simulink model "collagenSim"  (R2021b)
settings: Solver=VariableStepAuto  StartTime=0.0  StopTime=900  RelTol=1e-3
libraries: fl_lib x360, nesl_utility x174, rllib x1
(part 1 of 4)
settings Model: SimulationMode=accelerator  Creator=Genis  LastModifiedBy=Genis
settings SolverCC: ZeroCrossAlgorithm=Adaptive  DecoupledContinuousIntegration=on
settings DebuggingCC: ReadBeforeWriteMsg=DisableAll  WriteAfterWriteMsg=DisableAll  WriteAfterReadMsg=DisableAll  IgnoredZcDiagnostic=none  MultiTaskDSMMsg=none  UnitsInconsistencyMsg=none
settings ModelReferenceCC: UpdateModelReferenceTargets=IfOutOfDate
settings SFSimCC: SFSimEcho=off

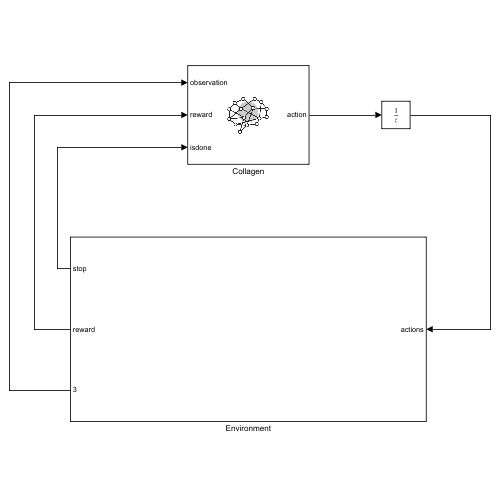
[thumbnail: Simulink's stored preview of the top-level diagram]
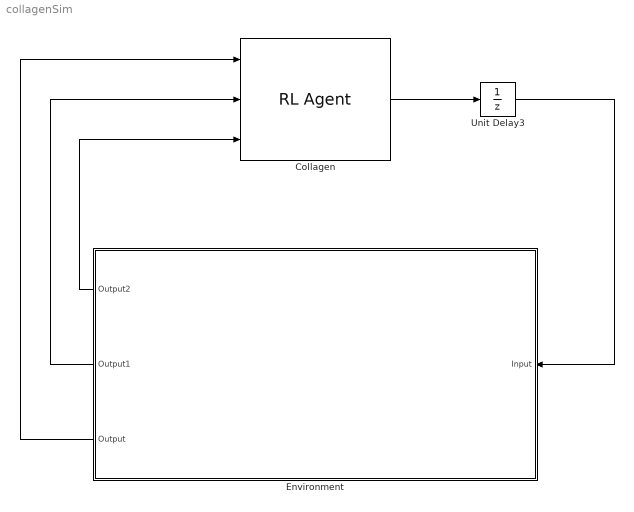
== system collagenSim ==
  Collagen : rllib/RL Agent  Agent=agent  ExternalActionAsInput=off  ProvideCumRwd=off  TreatAsDirectFeedthrough=on
  Environment : Subsystem
  Unit Delay3 : UnitDelay  InitialCondition=0.5*ones(15,1)  SampleTime=-1  HasFrameUpgradeWarning=on
  wires:
  Collagen/1 -> Unit Delay3/1
  Environment/1(Output2) -> Collagen/3
  Environment/2(Output1) -> Collagen/2
  Environment/3(Output) -> Collagen/1
  Unit Delay3/1 -> Environment/1(Input)

== system collagenSim/Environment ==
  Input : Inport
  Addition : MATLAB Function  TreatAsAtomicUnit=on
  Addition1 : MATLAB Function  TreatAsAtomicUnit=on
  Calculate Reward : MATLAB Function  TreatAsAtomicUnit=on
  Data center : Subsystem
  Demux : Demux  Outputs=15
  Incoming workloads : Subsystem
  Mux : Mux  Inputs=2
  Mux1 : Mux  Inputs=14
  Normalizer : Gain  Gain=1/348.15
  Rate Limiter : RateLimiter  RisingSlewLimit=0.15  FallingSlewLimit=-0.15  SampleTimeMode=inherited
  Scope{,1,4,6} (4 alike) : Scope
  Scope2 : Scope  NumInputPorts=2
  Scope3 : Scope  NumInputPorts=2
  Scope5 : Scope  NumInputPorts=2
  Output2 : Outport
  Output1 : Outport  Port=2
  Output : Outport  Port=3
  wires:
  Demux/3 -> Mux1/2
  Calculate Reward/2(stop) -> Output2/1, Scope3/2  "stop"
  Data center/4(Output1) -> Scope1/1, Addition/1(u)
  Calculate Reward/1(reward) -> Output1/1, Scope3/1  "reward"
  Data center/3(Output3) -> Calculate Reward/2(pwC), Addition1/1(u)
  Addition1/1(y) -> Scope2/1  "total cooling consumption"
  Addition/1(y) -> Scope2/2  "total operational consumption"
  Data center/1(Output) -> Mux/2, Scope/1, Calculate Reward/1(temps)
  Mux1/1 -> Data center/3(Input1)
  Demux/2 -> Mux1/1
  Data center/2(Output2) -> Scope6/1, Mux/1
  Demux/4 -> Mux1/3
  Demux/1 -> Data center/2(Input2)
  Demux/5 -> Mux1/4
  Mux/1 -> Normalizer/1  "env"
  Incoming workloads/1(Output) -> Data center/1(Input)
  Input/1 -> Rate Limiter/1, Scope5/1  "actions"
  Rate Limiter/1 -> Scope5/2, Demux/1
  Normalizer/1 -> Scope4/1, Output/1
  Demux/6 -> Mux1/5
  Demux/7 -> Mux1/6
  Demux/8 -> Mux1/7
  Demux/9 -> Mux1/8
  Demux/10 -> Mux1/9
  Demux/11 -> Mux1/10
  Demux/12 -> Mux1/11
  Demux/13 -> Mux1/12
  Demux/14 -> Mux1/13
  Demux/15 -> Mux1/14

== system collagenSim/Environment/Data center ==
  Input : Inport
  Input2 : Inport  Port=2
  Input1 : Inport  Port=3
  AC units : Subsystem
  Absolute Reference (MA) : fl_lib/Moist Air/Elements/Absolute Reference (MA)
      settings: SourceProductBaseCode=SS
  Absolute Reference (MA)1 : fl_lib/Moist Air/Elements/Absolute Reference (MA)
      settings: SourceProductBaseCode=SS
  Cabinet row 2 : Subsystem
      settings: PortSchema="{\"entries\":[{\"content\":{\"sides\":[{\"content\":{\"connectorIds\":[\"LConn1\",\"In1\",\"In2\",\"LConn2\"]},\"type\":\"ConnectorPlacement.EquallySpacedRectSide\",\"uuid\":\"aa64181a-7978-412f-98e9-dcdd97a3c7e3\"},{\"content\":{\"connectorIds\":[\"Out1\",\"Out2\",\"Out3\"],\"side\":\"RIGHT\"},\"type\":\"ConnectorPlacement.EquallySpacedRectSide\",\"uuid\":\"260fc92a-b2f9-43e3-aafe-e10e980a8ffc\"},{\"content\":{\"connectorIds\":[],\"side\":\"TOP\"},\"type\":\"ConnectorPlacement.EquallySpacedRectSide\",\"uuid\":\"89e14506-2648-4f30-8ee1-ca250c4b4586\"}]},\"type\":\"ConnectorPlacement.EquallySpacedConnector\",\"uuid\":\"d7223c8c-6a22-4f4f-a673-be755b2871a8\"}],\"packageUris\":[\"http://schema.mathworks.com/mf0/Connector/R2020b\"],\"version\":\"1.0\"}"
  Cabinet row 3 : Subsystem
      settings: PortSchema="{\"entries\":[{\"content\":{\"sides\":[{\"content\":{\"connectorIds\":[\"LConn1\",\"In1\",\"In2\",\"LConn2\"]},\"type\":\"ConnectorPlacement.EquallySpacedRectSide\",\"uuid\":\"aa64181a-7978-412f-98e9-dcdd97a3c7e3\"},{\"content\":{\"connectorIds\":[\"Out1\",\"Out2\",\"Out3\"],\"side\":\"RIGHT\"},\"type\":\"ConnectorPlacement.EquallySpacedRectSide\",\"uuid\":\"260fc92a-b2f9-43e3-aafe-e10e980a8ffc\"},{\"content\":{\"connectorIds\":[],\"side\":\"TOP\"},\"type\":\"ConnectorPlacement.EquallySpacedRectSide\",\"uuid\":\"89e14506-2648-4f30-8ee1-ca250c4b4586\"}]},\"type\":\"ConnectorPlacement.EquallySpacedConnector\",\"uuid\":\"d7223c8c-6a22-4f4f-a673-be755b2871a8\"}],\"packageUris\":[\"http://schema.mathworks.com/mf0/Connector/R2020b\"],\"version\":\"1.0\"}"
  Demux1 : Demux  Outputs=2
  Demux2 : Demux  Outputs=2
  Mux : Mux  Inputs=2
  Mux1 : Mux  Inputs=2
  Mux3 : Mux  Inputs=3
  PS-Simulink Converter{,1..3} (4 alike) : nesl_utility/PS-Simulink Converter  PhysicalDomain=network_engine_domain  SubClassName=ps_output  LeftPortType=input  RightPortType=output  PseudoPeriodic=off  Frequencies=[]  Unit=inherit  AffineConversion=off
      settings: SourceProductBaseCode=PW,SS
  Pressure & Temperature Sensor (MA) : fl_lib/Moist Air/Sensors/Pressure & Temperature Sensor (MA)
      settings: SourceProductBaseCode=SS  InternalSimscapePortConfiguration="{\"Bottom\":[],\"Left\":[{\"id\":\"A\",\"label\":\"A\",\"type\":\"foundation.moist_air.moist_air\"}],\"Right\":[{\"id\":\"B\",\"label\":\"B\",\"type\":\"foundation.moist_air.moist_air\"},{\"id\":\"P\",\"label\":\"P\",\"type\":\"output\"},{\"id\":\"T\",\"label\":\"T\",\"type\":\"output\"}],\"Top\":[]}"
  Pressure & Temperature Sensor (MA)1 : fl_lib/Moist Air/Sensors/Pressure & Temperature Sensor (MA)
      settings: SourceProductBaseCode=SS  InternalSimscapePortConfiguration="{\"Bottom\":[],\"Left\":[{\"id\":\"A\",\"label\":\"A\",\"type\":\"foundation.moist_air.moist_air\"}],\"Right\":[{\"id\":\"B\",\"label\":\"B\",\"type\":\"foundation.moist_air.moist_air\"},{\"id\":\"P\",\"label\":\"P\",\"type\":\"output\"},{\"id\":\"T\",\"label\":\"T\",\"type\":\"output\"}],\"Top\":[]}"
  Raised Floor : fl_lib/Moist Air/Elements/Constant Volume Chamber (MA)  volume=91.1*0.64 m^3  num_ports=foundation.enum.num_ports.two  area_A=2*0.6*0.9 m^2  area_B=4*(2*0.8*0.45+2*0.8*0.1) m^2  area_C=0.01 m^2  area_D=0.01 m^2  RH_ws=1  time_constant=1e-3 s  moisture_trace_gas_source=foundation.enum.moisture_trace_gas_source.none  moisture_source_spec=foundation.enum.moisture_source_spec.vapor  moisture_mass_flow=0 kg/s  moisture_temperature_spec=foundation.enum.temperature_spec.atmospheric  moisture_temperature=293.15 K  trace_gas_mass_flow=0 kg/s  trace_gas_temperature_spec=foundation.enum.temperature_spec.atmospheric  trace_gas_temperature=293.15 K  p_I_specify=off  p_I_priority=High  p_I=0.101325 MPa  p_I_nominal_specify=off  p_I_nominal_unit=MPa  p_I_nominal_value=1  T_I_specify=off  T_I_priority=High  T_I=293.15 K  T_I_nominal_specify=off  T_I_nominal_unit=K  T_I_nominal_value=1  RH_I_specify=off  RH_I_priority=High  RH_I=0  RH_I_nominal_specify=off  RH_I_nominal_unit=1  RH_I_nominal_value=1  x_w_I_specify=off  x_w_I_priority=None  x_w_I=0  x_w_I_nominal_specify=off  x_w_I_nominal_unit=1  x_w_I_nominal_value=1  y_w_I_specify=off  y_w_I_priority=None  y_w_I=0  y_w_I_nominal_specify=off  y_w_I_nominal_unit=1  y_w_I_nominal_value=1  HR_I_specify=off  HR_I_priority=None  HR_I=0  HR_I_nominal_specify=off  HR_I_nominal_unit=1  HR_I_nominal_value=1  x_g_I_specify=off  x_g_I_priority=High  x_g_I=0  x_g_I_nominal_specify=off  x_g_I_nominal_unit=1  x_g_I_nominal_value=1  y_g_I_specify=off  y_g_I_priority=None  y_g_I=0  y_g_I_nominal_specify=off  y_g_I_nominal_unit=1  y_g_I_nominal_value=1
      settings: SourceProductBaseCode=SS  InternalSimscapePortConfiguration="{\"Bottom\":[],\"Left\":[{\"id\":\"A\",\"label\":\"A\",\"type\":\"foundation.moist_air.moist_air\"},{\"id\":\"B\",\"label\":\"B\",\"type\":\"foundation.moist_air.moist_air\"}],\"Right\":[{\"id\":\"W\",\"label\":\"W\",\"type\":\"output\"},{\"id\":\"F\",\"label\":\"F\",\"type\":\"output\"},{\"id\":\"H\",\"label\":\"H\",\"type\":\"foundation.thermal.thermal\"}],\"Top\":[]}"
  Return : fl_lib/Moist Air/Elements/Local Restriction (MA)  restriction_type=foundation.enum.restriction_type.fixed  restriction_area=4*0.9 m^2  min_area=1e-10 m^2  max_area=0.005 m^2  area=4 m^2  Cd=0.64  B_lam=0.999
      settings: SourceProductBaseCode=SS  InternalSimscapePortConfiguration="{\"Bottom\":[],\"Left\":[{\"id\":\"A\",\"label\":\"A\",\"type\":\"foundation.moist_air.moist_air\"}],\"Right\":[{\"id\":\"B\",\"label\":\"B\",\"type\":\"foundation.moist_air.moist_air\"}],\"Top\":[]}"
  Rooom volume : fl_lib/Moist Air/Elements/Constant Volume Chamber (MA)  volume=91.1*4.5/2 m^3  num_ports=foundation.enum.num_ports.two  area_A=4*(2*0.8*0.45+2*0.8*0.1) m^2  area_B=2*0.6*0.9 m^2  area_C=0.01 m^2  area_D=0.01 m^2  RH_ws=1  time_constant=1e-3 s  moisture_trace_gas_source=foundation.enum.moisture_trace_gas_source.none  moisture_source_spec=foundation.enum.moisture_source_spec.vapor  moisture_mass_flow=0 kg/s  moisture_temperature_spec=foundation.enum.temperature_spec.atmospheric  moisture_temperature=293.15 K  trace_gas_mass_flow=0 kg/s  trace_gas_temperature_spec=foundation.enum.temperature_spec.atmospheric  trace_gas_temperature=293.15 K  p_I_specify=off  p_I_priority=High  p_I=0.101325 MPa  p_I_nominal_specify=off  p_I_nominal_unit=MPa  p_I_nominal_value=1  T_I_specify=off  T_I_priority=High  T_I=293.15 K  T_I_nominal_specify=off  T_I_nominal_unit=K  T_I_nominal_value=1  RH_I_specify=off  RH_I_priority=High  RH_I=0  RH_I_nominal_specify=off  RH_I_nominal_unit=1  RH_I_nominal_value=1  x_w_I_specify=off  x_w_I_priority=None  x_w_I=0  x_w_I_nominal_specify=off  x_w_I_nominal_unit=1  x_w_I_nominal_value=1  y_w_I_specify=off  y_w_I_priority=None  y_w_I=0  y_w_I_nominal_specify=off  y_w_I_nominal_unit=1  y_w_I_nominal_value=1  HR_I_specify=off  HR_I_priority=None  HR_I=0  HR_I_nominal_specify=off  HR_I_nominal_unit=1  HR_I_nominal_value=1  x_g_I_specify=off  x_g_I_priority=High  x_g_I=0  x_g_I_nominal_specify=off  x_g_I_nominal_unit=1  x_g_I_nominal_value=1  y_g_I_specify=off  y_g_I_priority=None  y_g_I=0  y_g_I_nominal_specify=off  y_g_I_nominal_unit=1  y_g_I_nominal_value=1
      settings: SourceProductBaseCode=SS  InternalSimscapePortConfiguration="{\"Bottom\":[],\"Left\":[{\"id\":\"A\",\"label\":\"A\",\"type\":\"foundation.moist_air.moist_air\"},{\"id\":\"B\",\"label\":\"B\",\"type\":\"foundation.moist_air.moist_air\"}],\"Right\":[{\"id\":\"W\",\"label\":\"W\",\"type\":\"output\"},{\"id\":\"F\",\"label\":\"F\",\"type\":\"output\"},{\"id\":\"H\",\"label\":\"H\",\"type\":\"foundation.thermal.thermal\"}],\"Top\":[]}"
  Scope : Scope
  Scope1 : Scope  NumInputPorts=2
  Scope2 : Scope
  Scope3 : Scope  NumInputPorts=2
  Scope5 : Scope
  Solver Configuration : nesl_utility/Solver Configuration  PhysicalDomain=network_engine_domain  SubClassName=solver  LeftPortType=input  RightPortType=generic  Tones=[]  Harmonics=[]  SimulateNoise=off  Profile=off  UseLocalSampling=off  EnableSwitchedLinearOptims=on  FrequencyDomain=off  UseCCode=off  RelTol=0.001  AbsTol=1e-06  MinStep=1e-09  ToWorkspace=off  RevertToSquareIcSolve=off  NumHomotopyIterations=100  PhasorMode=off  PhasorModeNumHarmonics=1  DoDC=off  ResidualTolerance=1e-09  UseLocalSolver=off  LocalSolverChoice=NE_BACKWARD_EULER_ADVANCER  LocalSolverSampleTime=0.001  DoFixedCost=off  MaxNonlinIter=3  MaxModeIter=2  ComputeImpulses=off  ImpulseIterations=2  LinearAlgebra=auto  EquationFormulation=NE_TIME_EF  DelaysMemoryBudget=1024  AutomaticFiltering=on  FilteringTimeConstant=0.001  PartitionStorageMethod=AS_NEEDED  PartitionMemoryBudget=1024  PartitionMethod=ROBUST
      settings: SourceProductBaseCode=PW,SS
  Output : Outport
  Output2 : Outport  Port=2
  Output3 : Outport  Port=3
  Output1 : Outport  Port=4
  wires:
  PS-Simulink Converter/1 -> Output2/1, Scope1/2  "room temperature"
  PS-Simulink Converter1/1 -> Scope1/1  "room pressure"
  Mux/1 -> Output/1, Scope/1  "server temperatures"
  PS-Simulink Converter3/1 -> Scope3/1  "floor pressure"
  PS-Simulink Converter2/1 -> Scope3/2  "floor temperature"
  Input/1 -> Demux1/1  "demands"
  Demux2/2 -> Cabinet row 2/2(fan speeds)
  Demux2/1 -> Cabinet row 3/2(fan speeds)
  Input1/1 -> Demux2/1  "fan speeds"
  Input2/1 -> AC units/1(Cooling)  "ac intensity"
  Mux1/1 -> Output1/1, Scope2/1  "server operational powers"
  Mux3/1 -> Output3/1, Scope5/1  "server cooling powers"
  Cabinet row 3/1(Out5) -> Mux/1  "temperatures"
  Cabinet row 2/1(Out5) -> Mux/2  "temperatures"
  Cabinet row 3/2(Out1) -> Mux1/1  "operational powers"
  Cabinet row 2/2(Out1) -> Mux1/2  "operational powers"
  Cabinet row 2/3(Out2) -> Mux3/3  "fan powers"
  Demux1/2 -> Cabinet row 3/1(demands)
  Demux1/1 -> Cabinet row 2/1(demands)
  AC units/1(cooling power) -> Mux3/1  "cooling power"
  Cabinet row 3/3(Out2) -> Mux3/2  "cooling power"
  connections:
  Rooom volume/LConn1 -- Cabinet row 2/LConn1 -- Cabinet row 3/LConn1 -- Return/RConn1 -- Pressure & Temperature Sensor (MA)/LConn1
  Rooom volume/LConn2 -- Solver Configuration/RConn1 -- AC units/LConn1
  Absolute Reference (MA)/LConn1 -- Pressure & Temperature Sensor (MA)/RConn1
  AC units/RConn1 -- Raised Floor/LConn1
  Cabinet row 3/LConn2 -- Return/LConn1 -- Raised Floor/LConn2 -- Cabinet row 2/LConn2 -- Pressure & Temperature Sensor (MA)1/LConn1
  PS-Simulink Converter/LConn1 -- Pressure & Temperature Sensor (MA)/RConn3
  PS-Simulink Converter1/LConn1 -- Pressure & Temperature Sensor (MA)/RConn2
  PS-Simulink Converter3/LConn1 -- Pressure & Temperature Sensor (MA)1/RConn2
  Absolute Reference (MA)1/LConn1 -- Pressure & Temperature Sensor (MA)1/RConn1
  PS-Simulink Converter2/LConn1 -- Pressure & Temperature Sensor (MA)1/RConn3

== system collagenSim/Environment/Incoming workloads ==
  Mux : Mux  Inputs=7
  Mux1 : Mux  Inputs=7
  Mux4 : Mux  Inputs=2
  Product{,1..13} (14 alike) : Product
  Random Number{1..14} (14 alike) : RandomNumber  Mean=1  Variance=0.01  Seed=randi(1e15)  SampleTime=60*5
  Rate Limiter1 : RateLimiter  RisingSlewLimit=0.0001  FallingSlewLimit=-0.0001  SampleTimeMode=inherited
  Scope : Scope
  Sine Wave{,1..13} (14 alike) : Sin  Amplitude=0.3+0.15*rand  Bias=0.4+0.2*rand  Frequency=2*pi/3600/24  Phase=2*pi*rand  SampleTime=0
  Output : Outport
  wires:
  Sine Wave2/1 -> Product2/1
  Random Number4/1 -> Product4/2
  Product5/1 -> Mux/6
  Random Number7/1 -> Product6/2
  Random Number1/1 -> Product/2
  Product1/1 -> Mux/2
  Sine Wave6/1 -> Product6/1
  Sine Wave/1 -> Product/1
  Sine Wave4/1 -> Product4/1
  Random Number3/1 -> Product2/2
  Random Number5/1 -> Product3/2
  Sine Wave3/1 -> Product3/1
  Sine Wave5/1 -> Product5/1
  Product/1 -> Mux/1
  Random Number6/1 -> Product5/2
  Random Number2/1 -> Product1/2
  Sine Wave1/1 -> Product1/1
  Product3/1 -> Mux/4
  Product6/1 -> Mux/7
  Product4/1 -> Mux/5
  Product2/1 -> Mux/3
  Product8/1 -> Mux1/2
  Product13/1 -> Mux1/7
  Product10/1 -> Mux1/4
  Product11/1 -> Mux1/5
  Product9/1 -> Mux1/3
  Product12/1 -> Mux1/6
  Product7/1 -> Mux1/1
  Mux1/1 -> Mux4/2
  Mux/1 -> Mux4/1
  Mux4/1 -> Rate Limiter1/1
  Rate Limiter1/1 -> Scope/1, Output/1
  Random Number9/1 -> Product8/2
  Random Number14/1 -> Product13/2
  Random Number13/1 -> Product12/2
  Random Number11/1 -> Product11/2
  Random Number10/1 -> Product9/2
  Sine Wave10/1 -> Product10/1
  Sine Wave13/1 -> Product13/1
  Sine Wave11/1 -> Product11/1
  Sine Wave7/1 -> Product7/1
  Sine Wave12/1 -> Product12/1
  Sine Wave8/1 -> Product8/1
  Sine Wave9/1 -> Product9/1
  Random Number8/1 -> Product7/2
  Random Number12/1 -> Product10/2

== system collagenSim/Environment/Data center/AC units ==
  note: There are 4 ac units in the room with a maximum energy consumption of 60 KW each, usually running at 19 KW, with a fan flow rate of 3.6 m^3/s. We have simplified this system by treating the fans and the air compression systems as one.
  Cooling : Inport
  AC units : fl_lib/Moist Air/Elements/Pipe (MA)  length=2 m  area=4/2 m^2  Dh=0.1 m  length_add=0.1 m  roughness=15e-6 m  Re_lam=2000  Re_tur=4000  shape_factor=64  Nu_lam=3.66  RH_ws=1  time_constant=1e-3 s  moisture_trace_gas_source=foundation.enum.moisture_trace_gas_source.none  moisture_source_spec=foundation.enum.moisture_source_spec.vapor  moisture_mass_flow=0 kg/s  moisture_temperature_spec=foundation.enum.temperature_spec.atmospheric  moisture_temperature=293.15 K  trace_gas_mass_flow=0 kg/s  trace_gas_temperature_spec=foundation.enum.temperature_spec.atmospheric  trace_gas_temperature=293.15 K  p_I_specify=off  p_I_priority=High  p_I=0.101325 MPa  p_I_nominal_specify=off  p_I_nominal_unit=MPa  p_I_nominal_value=1  T_I_specify=off  T_I_priority=High  T_I=293.15 K  T_I_nominal_specify=off  T_I_nominal_unit=K  T_I_nominal_value=1  RH_I_specify=off  RH_I_priority=High  RH_I=0  RH_I_nominal_specify=off  RH_I_nominal_unit=1  RH_I_nominal_value=1  x_w_I_specify=off  x_w_I_priority=None  x_w_I=0  x_w_I_nominal_specify=off  x_w_I_nominal_unit=1  x_w_I_nominal_value=1  y_w_I_specify=off  y_w_I_priority=None  y_w_I=0  y_w_I_nominal_specify=off  y_w_I_nominal_unit=1  y_w_I_nominal_value=1  HR_I_specify=off  HR_I_priority=None  HR_I=0  HR_I_nominal_specify=off  HR_I_nominal_unit=1  HR_I_nominal_value=1  x_g_I_specify=off  x_g_I_priority=High  x_g_I=0  x_g_I_nominal_specify=off  x_g_I_nominal_unit=1  x_g_I_nominal_value=1  y_g_I_specify=off  y_g_I_priority=None  y_g_I=0  y_g_I_nominal_specify=off  y_g_I_nominal_unit=1  y_g_I_nominal_value=1
      settings: SourceProductBaseCode=SS
  Controlled Volumetric Flow Rate Source (MA) : fl_lib/Moist Air/Sources/Controlled Volumetric Flow Rate Source (MA)  power_spec=foundation.enum.power_spec.isentropic  volumetric_flow_conditions=foundation.enum.volumetric_flow_conditions.actual  p_std=0.101325 MPa  T_std=20 degC  RH_std=0.65  area_A=2*0.6*0.9 m^2  area_B=2*0.6*0.9 m^2
      settings: SourceProductBaseCode=SS  InternalSimscapePortConfiguration="{\"Bottom\":[],\"Left\":[{\"id\":\"A\",\"label\":\"A\",\"type\":\"foundation.moist_air.moist_air\"},{\"id\":\"V\",\"label\":\"V\",\"type\":\"input\"}],\"Right\":[{\"id\":\"B\",\"label\":\"B\",\"type\":\"foundation.moist_air.moist_air\"}],\"Top\":[]}"
  Gain : Gain  Gain=3.6/19000
  Gain1 : Gain  Gain=2*60000
  Saturation : Saturate  UpperLimit=1  LowerLimit=0
  Simulink-PS Converter : nesl_utility/Simulink-PS Converter  PhysicalDomain=network_engine_domain  SubClassName=ps_input  LeftPortType=input  RightPortType=output  PseudoPeriodic=off  Frequencies=[]  NoiseDistribution=none  NoiseParameters=[]  Unit=1  AffineConversion=off  FilteringAndDerivatives=provide  SimscapeFilterOrder=1  InputFilterTimeConstant=0.001  UdotUserProvided=0
      settings: SourceProductBaseCode=PW,SS
  Temperature Source : fl_lib/Thermal/Thermal Sources/Temperature Source  temperature=12 degC
  Intake : PMIOPort  Side=Left
  Exhaust : PMIOPort  Port=2  Side=Right
  cooling power : Outport
  wires:
  Cooling/1 -> Saturation/1
  Gain1/1 -> cooling power/1, Gain/1
  Gain/1 -> Simulink-PS Converter/1
  Saturation/1 -> Gain1/1
  connections:
  Intake/RConn1 -- Controlled Volumetric Flow Rate Source (MA)/LConn1
  Simulink-PS Converter/RConn1 -- Controlled Volumetric Flow Rate Source (MA)/LConn2
  AC units/LConn1 -- Controlled Volumetric Flow Rate Source (MA)/RConn1
  Temperature Source/LConn1 -- AC units/LConn2
  AC units/RConn1 -- Exhaust/RConn1

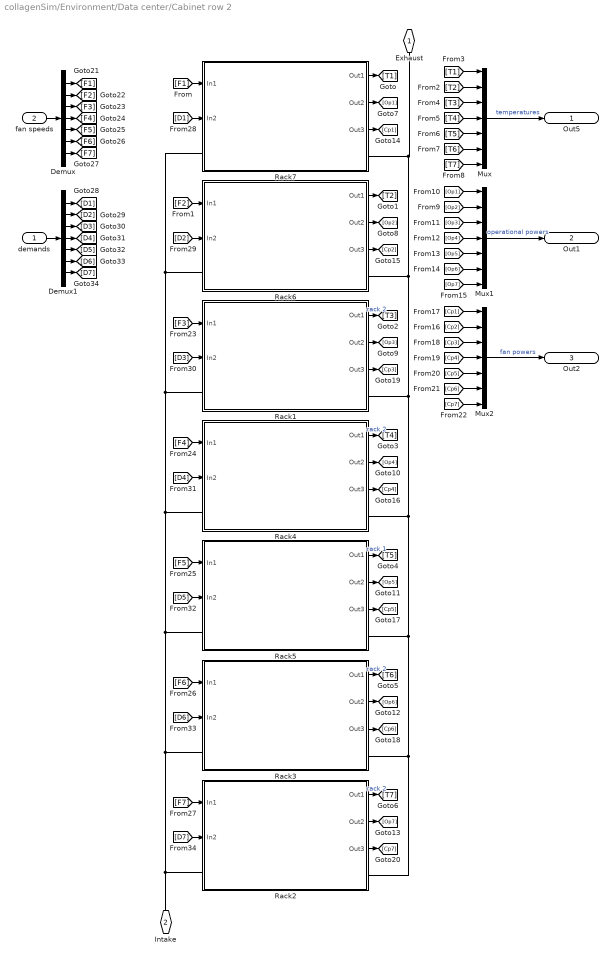
== system collagenSim/Environment/Data center/Cabinet row 2 ==
  demands : Inport
  fan speeds : Inport  Port=2
  Demux : Demux  Outputs=7
  Demux1 : Demux  Outputs=7
  Mux : Mux  Inputs=7
  Mux1 : Mux  Inputs=7
  Mux2 : Mux  Inputs=7
  Rack1 : Subsystem
  Rack2 : Subsystem
  Rack3 : Subsystem
  Rack4 : Subsystem
  Rack5 : Subsystem
  Rack6 : Subsystem
  Rack7 : Subsystem
  Exhaust : PMIOPort  Side=Left
  Intake : PMIOPort  Port=2  Side=Left
  Out5 : Outport
  Out1 : Outport  Port=2
  Out2 : Outport  Port=3
  wires:
  Mux/1 -> Out5/1  "temperatures"
  [T1] -> Mux/1
  Rack7/1(Out1) -> [T1]
  Rack6/1(Out1) -> [T2]
  [T2] -> Mux/2
  Rack1/1(Out1) -> [T3]  "rack 2"
  Rack2/1(Out1) -> [T7]  "rack 2"
  Rack3/1(Out1) -> [T6]  "rack 2"
  Rack5/1(Out1) -> [T5]  "rack 1"
  Rack4/1(Out1) -> [T4]  "rack 2"
  [T3] -> Mux/3
  [T4] -> Mux/4
  [T5] -> Mux/5
  [T6] -> Mux/6
  [T7] -> Mux/7
  Mux1/1 -> Out1/1  "operational powers"
  [Op5] -> Mux1/5
  [Op1] -> Mux1/1
  [Op2] -> Mux1/2
  [Op7] -> Mux1/7
  [Op6] -> Mux1/6
  [Op3] -> Mux1/3
  [Op4] -> Mux1/4
  Mux2/1 -> Out2/1  "fan powers"
  [Cp5] -> Mux2/5
  [Cp1] -> Mux2/1
  [Cp2] -> Mux2/2
  [Cp7] -> Mux2/7
  [Cp6] -> Mux2/6
  [Cp3] -> Mux2/3
  [Cp4] -> Mux2/4
  Rack7/2(Out2) -> [Op1]
  Rack6/2(Out2) -> [Op2]
  Rack1/2(Out2) -> [Op3]
  Rack4/2(Out2) -> [Op4]
  Rack5/2(Out2) -> [Op5]
  Rack3/2(Out2) -> [Op6]
  Rack2/2(Out2) -> [Op7]
  Rack7/3(Out3) -> [Cp1]
  Rack2/3(Out3) -> [Cp7]
  Rack3/3(Out3) -> [Cp6]
  Rack5/3(Out3) -> [Cp5]
  Rack4/3(Out3) -> [Cp4]
  Rack1/3(Out3) -> [Cp3]
  Rack6/3(Out3) -> [Cp2]
  Demux/1 -> [F1]
  Demux/2 -> [F2]
  Demux/3 -> [F3]
  Demux/4 -> [F4]
  Demux/5 -> [F5]
  Demux/6 -> [F6]
  Demux/7 -> [F7]
  Demux1/1 -> [D1]
  demands/1 -> Demux1/1
  fan speeds/1 -> Demux/1
  Demux1/2 -> [D2]
  Demux1/3 -> [D3]
  Demux1/4 -> [D4]
  Demux1/5 -> [D5]
  Demux1/6 -> [D6]
  Demux1/7 -> [D7]
  [F1] -> Rack7/1(In1)
  [F2] -> Rack6/1(In1)
  [F4] -> Rack4/1(In1)
  [F5] -> Rack5/1(In1)
  [F6] -> Rack3/1(In1)
  [F7] -> Rack2/1(In1)
  [D1] -> Rack7/2(In2)
  [D2] -> Rack6/2(In2)
  [D3] -> Rack1/2(In2)
  [D4] -> Rack4/2(In2)
  [D5] -> Rack5/2(In2)
  [D6] -> Rack3/2(In2)
  [D7] -> Rack2/2(In2)
  [F3] -> Rack1/1(In1)
  connections:
  Rack6/RConn1 -- Rack1/RConn1 -- Rack5/RConn1 -- Rack3/RConn1 -- Rack2/RConn1 -- Rack4/RConn1 -- Exhaust/RConn1 -- Rack7/RConn1
  Rack6/LConn1 -- Rack1/LConn1 -- Rack5/LConn1 -- Rack3/LConn1 -- Rack2/LConn1 -- Intake/RConn1 -- Rack4/LConn1 -- Rack7/LConn1

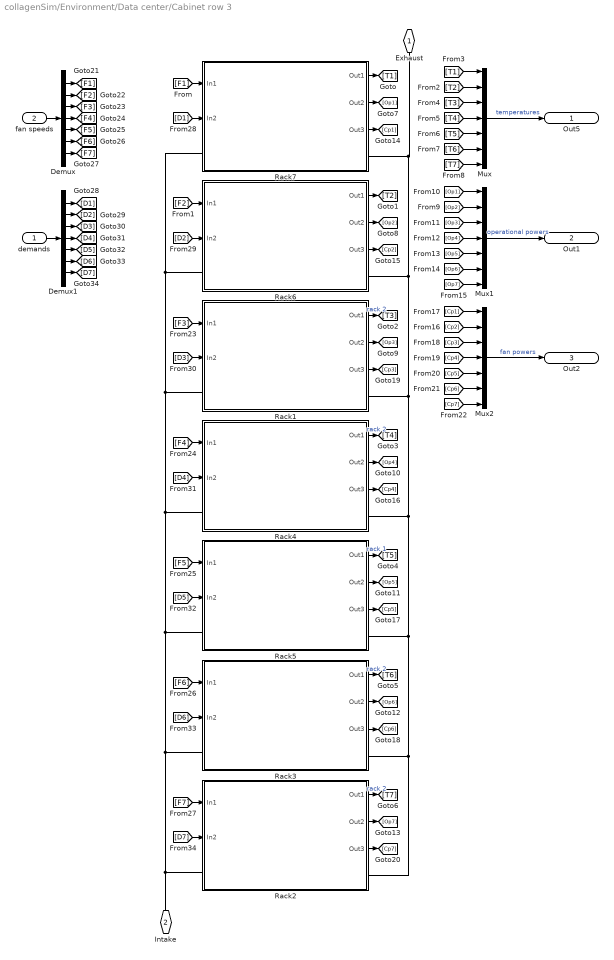
== system collagenSim/Environment/Data center/Cabinet row 3 ==
  demands : Inport
  fan speeds : Inport  Port=2
  Demux : Demux  Outputs=7
  Demux1 : Demux  Outputs=7
  Mux : Mux  Inputs=7
  Mux1 : Mux  Inputs=7
  Mux2 : Mux  Inputs=7
  Rack1 : Subsystem
  Rack2 : Subsystem
  Rack3 : Subsystem
  Rack4 : Subsystem
  Rack5 : Subsystem
  Rack6 : Subsystem
  Rack7 : Subsystem
  Exhaust : PMIOPort  Side=Left
  Intake : PMIOPort  Port=2  Side=Left
  Out5 : Outport
  Out1 : Outport  Port=2
  Out2 : Outport  Port=3
  wires:
  Mux/1 -> Out5/1  "temperatures"
  [T1] -> Mux/1
  Rack7/1(Out1) -> [T1]
  Rack6/1(Out1) -> [T2]
  [T2] -> Mux/2
  Rack1/1(Out1) -> [T3]  "rack 2"
  Rack2/1(Out1) -> [T7]  "rack 2"
  Rack3/1(Out1) -> [T6]  "rack 2"
  Rack5/1(Out1) -> [T5]  "rack 1"
  Rack4/1(Out1) -> [T4]  "rack 2"
  [T3] -> Mux/3
  [T4] -> Mux/4
  [T5] -> Mux/5
  [T6] -> Mux/6
  [T7] -> Mux/7
  Mux1/1 -> Out1/1  "operational powers"
  [Op5] -> Mux1/5
  [Op1] -> Mux1/1
  [Op2] -> Mux1/2
  [Op7] -> Mux1/7
  [Op6] -> Mux1/6
  [Op3] -> Mux1/3
  [Op4] -> Mux1/4
  Mux2/1 -> Out2/1  "fan powers"
  [Cp5] -> Mux2/5
  [Cp1] -> Mux2/1
  [Cp2] -> Mux2/2
  [Cp7] -> Mux2/7
  [Cp6] -> Mux2/6
  [Cp3] -> Mux2/3
  [Cp4] -> Mux2/4
  Rack7/2(Out2) -> [Op1]
  Rack6/2(Out2) -> [Op2]
  Rack1/2(Out2) -> [Op3]
  Rack4/2(Out2) -> [Op4]
  Rack5/2(Out2) -> [Op5]
  Rack3/2(Out2) -> [Op6]
  Rack2/2(Out2) -> [Op7]
  Rack7/3(Out3) -> [Cp1]
  Rack2/3(Out3) -> [Cp7]
  Rack3/3(Out3) -> [Cp6]
  Rack5/3(Out3) -> [Cp5]
  Rack4/3(Out3) -> [Cp4]
  Rack1/3(Out3) -> [Cp3]
  Rack6/3(Out3) -> [Cp2]
  Demux/1 -> [F1]
  Demux/2 -> [F2]
  Demux/3 -> [F3]
  Demux/4 -> [F4]
  Demux/5 -> [F5]
  Demux/6 -> [F6]
  Demux/7 -> [F7]
  Demux1/1 -> [D1]
  demands/1 -> Demux1/1
  fan speeds/1 -> Demux/1
  Demux1/2 -> [D2]
  Demux1/3 -> [D3]
  Demux1/4 -> [D4]
  Demux1/5 -> [D5]
  Demux1/6 -> [D6]
  Demux1/7 -> [D7]
  [F1] -> Rack7/1(In1)
  [F2] -> Rack6/1(In1)
  [F4] -> Rack4/1(In1)
  [F5] -> Rack5/1(In1)
  [F6] -> Rack3/1(In1)
  [F7] -> Rack2/1(In1)
  [D1] -> Rack7/2(In2)
  [D2] -> Rack6/2(In2)
  [D3] -> Rack1/2(In2)
  [D4] -> Rack4/2(In2)
  [D5] -> Rack5/2(In2)
  [D6] -> Rack3/2(In2)
  [D7] -> Rack2/2(In2)
  [F3] -> Rack1/1(In1)
  connections:
  Rack6/RConn1 -- Rack1/RConn1 -- Rack5/RConn1 -- Rack3/RConn1 -- Rack2/RConn1 -- Rack4/RConn1 -- Exhaust/RConn1 -- Rack7/RConn1
  Rack6/LConn1 -- Rack1/LConn1 -- Rack5/LConn1 -- Rack3/LConn1 -- Rack2/LConn1 -- Intake/RConn1 -- Rack4/LConn1 -- Rack7/LConn1

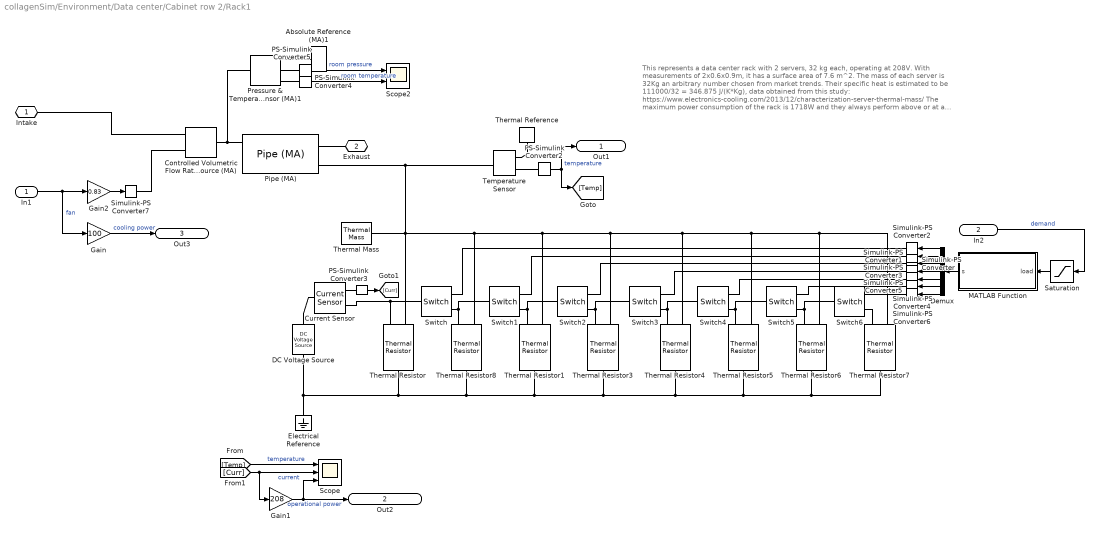
== system collagenSim/Environment/Data center/Cabinet row 2/Rack1 ==
  note: This represents a data center rack with 2 servers, 32 kg each, operating at 208V. With measurements of 2x0.6x0.9m, it has a surface area of 7.6 m^2. The mass of each server is 32Kg an arbitrary number chosen from market trends. Their specific heat is estimated to be 111000/32 = 346.875 J/(K*Kg), data obtained from this study: https://www.electronics-cooling.com/2013/12/characterization-server-thermal-mass/
      | The maximum power consumption of the rack is 1718W and they always perform above or at a minumum of 214.75W.
      | The rack's temperature exchange with the outside environment is modeled with a fluid pipe using the thermal propeties of air at sea level. The cooling system is modeled as eight 8mm four fan panels consuming a maximum of 100W per panel, which gives to each of the eight a total maximum vulumetric rate of 212m^3/min, meaning 0.83m^3/s. The surface area of the pipe representing the interior of the servers has been underestimated to be equal to the surface of the casing that contains them.
  In1 : Inport
  In2 : Inport  Port=2
  Absolute Reference (MA)1 : fl_lib/Moist Air/Elements/Absolute Reference (MA)
      settings: SourceProductBaseCode=SS
  Controlled Volumetric Flow Rate Source (MA) : fl_lib/Moist Air/Sources/Controlled Volumetric Flow Rate Source (MA)  power_spec=foundation.enum.power_spec.isentropic  volumetric_flow_conditions=foundation.enum.volumetric_flow_conditions.actual  p_std=0.101325 MPa  T_std=20 degC  RH_std=0.65  area_A=2*(2*0.442*0.4+2*0.442*0.711) m^2  area_B=2*(2*0.442*0.4+2*0.442*0.711) m^2
      settings: SourceProductBaseCode=SS  InternalSimscapePortConfiguration="{\"Bottom\":[],\"Left\":[{\"id\":\"A\",\"label\":\"A\",\"type\":\"foundation.moist_air.moist_air\"},{\"id\":\"V\",\"label\":\"V\",\"type\":\"input\"}],\"Right\":[{\"id\":\"B\",\"label\":\"B\",\"type\":\"foundation.moist_air.moist_air\"}],\"Top\":[]}"
  Current Sensor : fl_lib/Electrical/Electrical Sensors/Current Sensor
  DC Voltage Source : fl_lib/Electrical/Electrical Sources/DC Voltage Source  v0=208 V
  Demux : Demux  Outputs=7
  Electrical Reference : fl_lib/Electrical/Electrical Elements/Electrical Reference
  Gain : Gain  Gain=100
  Gain1 : Gain  Gain=208
  Gain2 : Gain  Gain=0.83
  MATLAB Function : MATLAB Function  TreatAsAtomicUnit=on
  PS-Simulink Converter{2..5} (4 alike) : nesl_utility/PS-Simulink Converter  PhysicalDomain=network_engine_domain  SubClassName=ps_output  LeftPortType=input  RightPortType=output  PseudoPeriodic=off  Frequencies=[]  Unit=inherit  AffineConversion=off
      settings: SourceProductBaseCode=PW,SS
  Pipe (MA) : fl_lib/Moist Air/Elements/Pipe (MA)  length=0.711 m  area=2*(2*0.442*0.4+2*0.442*0.711) m^2  Dh=0.1 m  length_add=0.1 m  roughness=15e-6 m  Re_lam=2000  Re_tur=4000  shape_factor=64  Nu_lam=3.66  RH_ws=1  time_constant=1e-3 s  moisture_trace_gas_source=foundation.enum.moisture_trace_gas_source.none  moisture_source_spec=foundation.enum.moisture_source_spec.vapor  moisture_mass_flow=0 kg/s  moisture_temperature_spec=foundation.enum.temperature_spec.atmospheric  moisture_temperature=293.15 K  trace_gas_mass_flow=0 kg/s  trace_gas_temperature_spec=foundation.enum.temperature_spec.atmospheric  trace_gas_temperature=293.15 K  p_I_specify=off  p_I_priority=High  p_I=0.101325 MPa  p_I_nominal_specify=off  p_I_nominal_unit=MPa  p_I_nominal_value=1  T_I_specify=off  T_I_priority=High  T_I=293.15 K  T_I_nominal_specify=off  T_I_nominal_unit=K  T_I_nominal_value=1  RH_I_specify=off  RH_I_priority=High  RH_I=0  RH_I_nominal_specify=off  RH_I_nominal_unit=1  RH_I_nominal_value=1  x_w_I_specify=off  x_w_I_priority=None  x_w_I=0  x_w_I_nominal_specify=off  x_w_I_nominal_unit=1  x_w_I_nominal_value=1  y_w_I_specify=off  y_w_I_priority=None  y_w_I=0  y_w_I_nominal_specify=off  y_w_I_nominal_unit=1  y_w_I_nominal_value=1  HR_I_specify=off  HR_I_priority=None  HR_I=0  HR_I_nominal_specify=off  HR_I_nominal_unit=1  HR_I_nominal_value=1  x_g_I_specify=off  x_g_I_priority=High  x_g_I=0  x_g_I_nominal_specify=off  x_g_I_nominal_unit=1  x_g_I_nominal_value=1  y_g_I_specify=off  y_g_I_priority=None  y_g_I=0  y_g_I_nominal_specify=off  y_g_I_nominal_unit=1  y_g_I_nominal_value=1
      settings: SourceProductBaseCode=SS
  Pressure & Temperature Sensor (MA)1 : fl_lib/Moist Air/Sensors/Pressure & Temperature Sensor (MA)
      settings: SourceProductBaseCode=SS  InternalSimscapePortConfiguration="{\"Bottom\":[],\"Left\":[{\"id\":\"A\",\"label\":\"A\",\"type\":\"foundation.moist_air.moist_air\"}],\"Right\":[{\"id\":\"B\",\"label\":\"B\",\"type\":\"foundation.moist_air.moist_air\"},{\"id\":\"P\",\"label\":\"P\",\"type\":\"output\"},{\"id\":\"T\",\"label\":\"T\",\"type\":\"output\"}],\"Top\":[]}"
  Saturation : Saturate  UpperLimit=0.99  LowerLimit=0.01
  Scope : Scope  NumInputPorts=3
  Scope2 : Scope  NumInputPorts=2
  Simulink-PS Converter{,1..7} (8 alike) : nesl_utility/Simulink-PS Converter  PhysicalDomain=network_engine_domain  SubClassName=ps_input  LeftPortType=input  RightPortType=output  PseudoPeriodic=off  Frequencies=[]  NoiseDistribution=none  NoiseParameters=[]  Unit=1  AffineConversion=off  FilteringAndDerivatives=provide  SimscapeFilterOrder=1  InputFilterTimeConstant=0.001  UdotUserProvided=0
      settings: SourceProductBaseCode=PW,SS
  Switch{,1..6} (7 alike) : fl_lib/Electrical/Electrical Elements/Switch  R_closed=0.01 Ohm  G_open=1e-8 1/Ohm  Threshold=0.5  i_specify=off  i_priority=None  i=0 A  i_nominal_specify=off  i_nominal_unit=A  i_nominal_value=1  v_specify=off  v_priority=None  v=0 V  v_nominal_specify=off  v_nominal_unit=V  v_nominal_value=1
  Temperature Sensor : fl_lib/Thermal/Thermal Sensors/Temperature Sensor
  Thermal Mass : fl_lib/Thermal/Thermal Elements/Thermal Mass  mass=64 kg  sp_heat=346.875 J/(K*kg)  T_specify=on  T_priority=High  T=293.15 K  T_nominal_specify=off  T_nominal_unit=K  T_nominal_value=1  Q_specify=off  Q_priority=None  Q=0 W  Q_nominal_specify=off  Q_nominal_unit=W  Q_nominal_value=1
  Thermal Reference : fl_lib/Thermal/Thermal Elements/Thermal Reference
  Thermal Resistor{,1,3..8} (8 alike) : fl_lib/Electrical/Electrical Elements/Thermal Resistor  R0=208^2/1718*8 Ohm  T0=298.15 K  alpha=50e-6 1/K  tc=10 s  K_d=1e-3 W/K  T_specify=on  T_priority=High  T=293.15 K  T_nominal_specify=off  T_nominal_unit=K  T_nominal_value=1
      settings: SourceProductBaseCode=SS  InternalSimscapePortConfiguration="{\"Bottom\":[],\"Left\":[{\"id\":\"H\",\"label\":\"H\",\"type\":\"foundation.thermal.thermal\"},{\"id\":\"p\",\"label\":\"+\",\"type\":\"foundation.electrical.electrical\"}],\"Right\":[{\"id\":\"n\",\"label\":\"-\",\"type\":\"foundation.electrical.electrical\"}],\"Top\":[]}"
  Intake : PMIOPort  Side=Left
  Exhaust : PMIOPort  Port=2  Side=Right
  Out1 : Outport
  Out2 : Outport  Port=2
  Out3 : Outport  Port=3
  wires:
  Demux/6 -> Simulink-PS Converter5/1
  Demux/1 -> Simulink-PS Converter2/1
  Demux/2 -> Simulink-PS Converter1/1
  Demux/7 -> Simulink-PS Converter6/1
  PS-Simulink Converter2/1 -> Out1/1, [Temp]  "temperature"
  [Curr] -> Scope/2, Gain1/1  "current"
  [Temp] -> Scope/1  "temperature"
  PS-Simulink Converter3/1 -> [Curr]
  Saturation/1 -> MATLAB Function/1(load)
  In2/1 -> Saturation/1  "demand"
  Demux/4 -> Simulink-PS Converter3/1
  Demux/3 -> Simulink-PS Converter/1
  Demux/5 -> Simulink-PS Converter4/1
  MATLAB Function/1(s) -> Demux/1
  Gain1/1 -> Out2/1, Scope/3  "operational power"
  In1/1 -> Gain/1, Gain2/1  "fan"
  Gain2/1 -> Simulink-PS Converter7/1
  Gain/1 -> Out3/1  "cooling power"
  PS-Simulink Converter5/1 -> Scope2/1  "room pressure"
  PS-Simulink Converter4/1 -> Scope2/2  "room temperature"
  connections:
  Switch3/LConn1 -- Switch2/RConn2 -- Thermal Resistor3/LConn2
  Thermal Resistor3/RConn1 -- Thermal Resistor6/RConn1 -- Thermal Resistor7/RConn1 -- Thermal Resistor5/RConn1 -- Thermal Resistor4/RConn1 -- Thermal Resistor8/RConn1 -- Electrical Reference/LConn1 -- DC Voltage Source/RConn1 -- Thermal Resistor/RConn1 -- Thermal Resistor1/RConn1
  DC Voltage Source/LConn1 -- Current Sensor/LConn1
  Switch2/LConn1 -- Switch1/RConn2 -- Thermal Resistor1/LConn2
  Switch1/LConn1 -- Switch/RConn2 -- Thermal Resistor8/LConn2
  Thermal Resistor4/LConn2 -- Switch4/LConn1 -- Switch3/RConn2
  Switch6/LConn1 -- Switch5/RConn2 -- Thermal Resistor6/LConn2
  Switch/LConn1 -- Current Sensor/RConn2 -- Thermal Resistor/LConn2
  Thermal Resistor5/LConn2 -- Switch5/LConn1 -- Switch4/RConn2
  Thermal Reference/LConn1 -- Temperature Sensor/RConn1
  Simulink-PS Converter6/RConn1 -- Switch6/RConn1
  Thermal Resistor7/LConn2 -- Switch6/RConn2
  Simulink-PS Converter4/RConn1 -- Switch4/RConn1
  Simulink-PS Converter2/RConn1 -- Switch/RConn1
  Simulink-PS Converter1/RConn1 -- Switch1/RConn1
  Temperature Sensor/RConn2 -- PS-Simulink Converter2/LConn1
  Simulink-PS Converter/RConn1 -- Switch2/RConn1
  Current Sensor/RConn1 -- PS-Simulink Converter3/LConn1
  Simulink-PS Converter3/RConn1 -- Switch3/RConn1
  Simulink-PS Converter5/RConn1 -- Switch5/RConn1
  Controlled Volumetric Flow Rate Source (MA)/LConn2 -- Simulink-PS Converter7/RConn1
  Pipe (MA)/RConn1 -- Controlled Volumetric Flow Rate Source (MA)/RConn1 -- Pressure & Temperature Sensor (MA)1/LConn1
  Intake/RConn1 -- Controlled Volumetric Flow Rate Source (MA)/LConn1
  Pipe (MA)/LConn1 -- Exhaust/RConn1
  Thermal Resistor8/LConn1 -- Pipe (MA)/LConn2 -- Temperature Sensor/LConn1 -- Thermal Resistor/LConn1 -- Thermal Mass/LConn1 -- Thermal Resistor6/LConn1 -- Thermal Resistor7/LConn1 -- Thermal Resistor5/LConn1 -- Thermal Resistor4/LConn1 -- Thermal Resistor3/LConn1 -- Thermal Resistor1/LConn1
  PS-Simulink Converter5/LConn1 -- Pressure & Temperature Sensor (MA)1/RConn2
  PS-Simulink Converter4/LConn1 -- Pressure & Temperature Sensor (MA)1/RConn3
  Absolute Reference (MA)1/LConn1 -- Pressure & Temperature Sensor (MA)1/RConn1

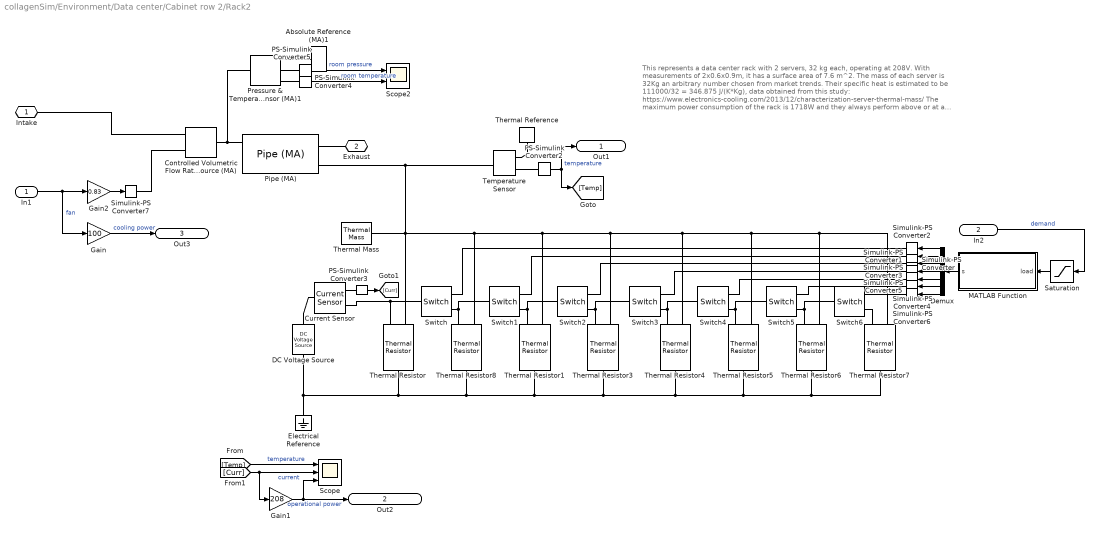
== system collagenSim/Environment/Data center/Cabinet row 2/Rack2 ==
  note: This represents a data center rack with 2 servers, 32 kg each, operating at 208V. With measurements of 2x0.6x0.9m, it has a surface area of 7.6 m^2. The mass of each server is 32Kg an arbitrary number chosen from market trends. Their specific heat is estimated to be 111000/32 = 346.875 J/(K*Kg), data obtained from this study: https://www.electronics-cooling.com/2013/12/characterization-server-thermal-mass/
      | The maximum power consumption of the rack is 1718W and they always perform above or at a minumum of 214.75W.
      | The rack's temperature exchange with the outside environment is modeled with a fluid pipe using the thermal propeties of air at sea level. The cooling system is modeled as eight 8mm four fan panels consuming a maximum of 100W per panel, which gives to each of the eight a total maximum vulumetric rate of 212m^3/min, meaning 0.83m^3/s. The surface area of the pipe representing the interior of the servers has been underestimated to be equal to the surface of the casing that contains them.
  In1 : Inport
  In2 : Inport  Port=2
  Absolute Reference (MA)1 : fl_lib/Moist Air/Elements/Absolute Reference (MA)
      settings: SourceProductBaseCode=SS
  Controlled Volumetric Flow Rate Source (MA) : fl_lib/Moist Air/Sources/Controlled Volumetric Flow Rate Source (MA)  power_spec=foundation.enum.power_spec.isentropic  volumetric_flow_conditions=foundation.enum.volumetric_flow_conditions.actual  p_std=0.101325 MPa  T_std=20 degC  RH_std=0.65  area_A=2*(2*0.442*0.4+2*0.442*0.711) m^2  area_B=2*(2*0.442*0.4+2*0.442*0.711) m^2
      settings: SourceProductBaseCode=SS  InternalSimscapePortConfiguration="{\"Bottom\":[],\"Left\":[{\"id\":\"A\",\"label\":\"A\",\"type\":\"foundation.moist_air.moist_air\"},{\"id\":\"V\",\"label\":\"V\",\"type\":\"input\"}],\"Right\":[{\"id\":\"B\",\"label\":\"B\",\"type\":\"foundation.moist_air.moist_air\"}],\"Top\":[]}"
  Current Sensor : fl_lib/Electrical/Electrical Sensors/Current Sensor
  DC Voltage Source : fl_lib/Electrical/Electrical Sources/DC Voltage Source  v0=208 V
  Demux : Demux  Outputs=7
  Electrical Reference : fl_lib/Electrical/Electrical Elements/Electrical Reference
  Gain : Gain  Gain=100
  Gain1 : Gain  Gain=208
  Gain2 : Gain  Gain=0.83
  MATLAB Function : MATLAB Function  TreatAsAtomicUnit=on
  PS-Simulink Converter{2..5} (4 alike) : nesl_utility/PS-Simulink Converter  PhysicalDomain=network_engine_domain  SubClassName=ps_output  LeftPortType=input  RightPortType=output  PseudoPeriodic=off  Frequencies=[]  Unit=inherit  AffineConversion=off
      settings: SourceProductBaseCode=PW,SS
  Pipe (MA) : fl_lib/Moist Air/Elements/Pipe (MA)  length=0.711 m  area=2*(2*0.442*0.4+2*0.442*0.711) m^2  Dh=0.1 m  length_add=0.1 m  roughness=15e-6 m  Re_lam=2000  Re_tur=4000  shape_factor=64  Nu_lam=3.66  RH_ws=1  time_constant=1e-3 s  moisture_trace_gas_source=foundation.enum.moisture_trace_gas_source.none  moisture_source_spec=foundation.enum.moisture_source_spec.vapor  moisture_mass_flow=0 kg/s  moisture_temperature_spec=foundation.enum.temperature_spec.atmospheric  moisture_temperature=293.15 K  trace_gas_mass_flow=0 kg/s  trace_gas_temperature_spec=foundation.enum.temperature_spec.atmospheric  trace_gas_temperature=293.15 K  p_I_specify=off  p_I_priority=High  p_I=0.101325 MPa  p_I_nominal_specify=off  p_I_nominal_unit=MPa  p_I_nominal_value=1  T_I_specify=off  T_I_priority=High  T_I=293.15 K  T_I_nominal_specify=off  T_I_nominal_unit=K  T_I_nominal_value=1  RH_I_specify=off  RH_I_priority=High  RH_I=0  RH_I_nominal_specify=off  RH_I_nominal_unit=1  RH_I_nominal_value=1  x_w_I_specify=off  x_w_I_priority=None  x_w_I=0  x_w_I_nominal_specify=off  x_w_I_nominal_unit=1  x_w_I_nominal_value=1  y_w_I_specify=off  y_w_I_priority=None  y_w_I=0  y_w_I_nominal_specify=off  y_w_I_nominal_unit=1  y_w_I_nominal_value=1  HR_I_specify=off  HR_I_priority=None  HR_I=0  HR_I_nominal_specify=off  HR_I_nominal_unit=1  HR_I_nominal_value=1  x_g_I_specify=off  x_g_I_priority=High  x_g_I=0  x_g_I_nominal_specify=off  x_g_I_nominal_unit=1  x_g_I_nominal_value=1  y_g_I_specify=off  y_g_I_priority=None  y_g_I=0  y_g_I_nominal_specify=off  y_g_I_nominal_unit=1  y_g_I_nominal_value=1
      settings: SourceProductBaseCode=SS
  Pressure & Temperature Sensor (MA)1 : fl_lib/Moist Air/Sensors/Pressure & Temperature Sensor (MA)
      settings: SourceProductBaseCode=SS  InternalSimscapePortConfiguration="{\"Bottom\":[],\"Left\":[{\"id\":\"A\",\"label\":\"A\",\"type\":\"foundation.moist_air.moist_air\"}],\"Right\":[{\"id\":\"B\",\"label\":\"B\",\"type\":\"foundation.moist_air.moist_air\"},{\"id\":\"P\",\"label\":\"P\",\"type\":\"output\"},{\"id\":\"T\",\"label\":\"T\",\"type\":\"output\"}],\"Top\":[]}"
  Saturation : Saturate  UpperLimit=0.99  LowerLimit=0.01
  Scope : Scope  NumInputPorts=3
  Scope2 : Scope  NumInputPorts=2
  Simulink-PS Converter{,1..7} (8 alike) : nesl_utility/Simulink-PS Converter  PhysicalDomain=network_engine_domain  SubClassName=ps_input  LeftPortType=input  RightPortType=output  PseudoPeriodic=off  Frequencies=[]  NoiseDistribution=none  NoiseParameters=[]  Unit=1  AffineConversion=off  FilteringAndDerivatives=provide  SimscapeFilterOrder=1  InputFilterTimeConstant=0.001  UdotUserProvided=0
      settings: SourceProductBaseCode=PW,SS
  Switch{,1..6} (7 alike) : fl_lib/Electrical/Electrical Elements/Switch  R_closed=0.01 Ohm  G_open=1e-8 1/Ohm  Threshold=0.5  i_specify=off  i_priority=None  i=0 A  i_nominal_specify=off  i_nominal_unit=A  i_nominal_value=1  v_specify=off  v_priority=None  v=0 V  v_nominal_specify=off  v_nominal_unit=V  v_nominal_value=1
  Temperature Sensor : fl_lib/Thermal/Thermal Sensors/Temperature Sensor
  Thermal Mass : fl_lib/Thermal/Thermal Elements/Thermal Mass  mass=64 kg  sp_heat=346.875 J/(K*kg)  T_specify=on  T_priority=High  T=293.15 K  T_nominal_specify=off  T_nominal_unit=K  T_nominal_value=1  Q_specify=off  Q_priority=None  Q=0 W  Q_nominal_specify=off  Q_nominal_unit=W  Q_nominal_value=1
  Thermal Reference : fl_lib/Thermal/Thermal Elements/Thermal Reference
  Thermal Resistor{,1,3..8} (8 alike) : fl_lib/Electrical/Electrical Elements/Thermal Resistor  R0=208^2/1718*8 Ohm  T0=298.15 K  alpha=50e-6 1/K  tc=10 s  K_d=1e-3 W/K  T_specify=on  T_priority=High  T=293.15 K  T_nominal_specify=off  T_nominal_unit=K  T_nominal_value=1
      settings: SourceProductBaseCode=SS  InternalSimscapePortConfiguration="{\"Bottom\":[],\"Left\":[{\"id\":\"H\",\"label\":\"H\",\"type\":\"foundation.thermal.thermal\"},{\"id\":\"p\",\"label\":\"+\",\"type\":\"foundation.electrical.electrical\"}],\"Right\":[{\"id\":\"n\",\"label\":\"-\",\"type\":\"foundation.electrical.electrical\"}],\"Top\":[]}"
  Intake : PMIOPort  Side=Left
  Exhaust : PMIOPort  Port=2  Side=Right
  Out1 : Outport
  Out2 : Outport  Port=2
  Out3 : Outport  Port=3
  wires:
  Demux/6 -> Simulink-PS Converter5/1
  Demux/1 -> Simulink-PS Converter2/1
  Demux/2 -> Simulink-PS Converter1/1
  Demux/7 -> Simulink-PS Converter6/1
  PS-Simulink Converter2/1 -> Out1/1, [Temp]  "temperature"
  [Curr] -> Scope/2, Gain1/1  "current"
  [Temp] -> Scope/1  "temperature"
  PS-Simulink Converter3/1 -> [Curr]
  Saturation/1 -> MATLAB Function/1(load)
  In2/1 -> Saturation/1  "demand"
  Demux/4 -> Simulink-PS Converter3/1
  Demux/3 -> Simulink-PS Converter/1
  Demux/5 -> Simulink-PS Converter4/1
  MATLAB Function/1(s) -> Demux/1
  Gain1/1 -> Out2/1, Scope/3  "operational power"
  In1/1 -> Gain/1, Gain2/1  "fan"
  Gain2/1 -> Simulink-PS Converter7/1
  Gain/1 -> Out3/1  "cooling power"
  PS-Simulink Converter5/1 -> Scope2/1  "room pressure"
  PS-Simulink Converter4/1 -> Scope2/2  "room temperature"
  connections:
  Switch3/LConn1 -- Switch2/RConn2 -- Thermal Resistor3/LConn2
  Thermal Resistor3/RConn1 -- Thermal Resistor6/RConn1 -- Thermal Resistor7/RConn1 -- Thermal Resistor5/RConn1 -- Thermal Resistor4/RConn1 -- Thermal Resistor8/RConn1 -- Electrical Reference/LConn1 -- DC Voltage Source/RConn1 -- Thermal Resistor/RConn1 -- Thermal Resistor1/RConn1
  DC Voltage Source/LConn1 -- Current Sensor/LConn1
  Switch2/LConn1 -- Switch1/RConn2 -- Thermal Resistor1/LConn2
  Switch1/LConn1 -- Switch/RConn2 -- Thermal Resistor8/LConn2
  Thermal Resistor4/LConn2 -- Switch4/LConn1 -- Switch3/RConn2
  Switch6/LConn1 -- Switch5/RConn2 -- Thermal Resistor6/LConn2
  Switch/LConn1 -- Current Sensor/RConn2 -- Thermal Resistor/LConn2
  Thermal Resistor5/LConn2 -- Switch5/LConn1 -- Switch4/RConn2
  Thermal Reference/LConn1 -- Temperature Sensor/RConn1
  Simulink-PS Converter6/RConn1 -- Switch6/RConn1
  Thermal Resistor7/LConn2 -- Switch6/RConn2
  Simulink-PS Converter4/RConn1 -- Switch4/RConn1
  Simulink-PS Converter2/RConn1 -- Switch/RConn1
  Simulink-PS Converter1/RConn1 -- Switch1/RConn1
  Temperature Sensor/RConn2 -- PS-Simulink Converter2/LConn1
  Simulink-PS Converter/RConn1 -- Switch2/RConn1
  Current Sensor/RConn1 -- PS-Simulink Converter3/LConn1
  Simulink-PS Converter3/RConn1 -- Switch3/RConn1
  Simulink-PS Converter5/RConn1 -- Switch5/RConn1
  Controlled Volumetric Flow Rate Source (MA)/LConn2 -- Simulink-PS Converter7/RConn1
  Pipe (MA)/RConn1 -- Controlled Volumetric Flow Rate Source (MA)/RConn1 -- Pressure & Temperature Sensor (MA)1/LConn1
  Intake/RConn1 -- Controlled Volumetric Flow Rate Source (MA)/LConn1
  Pipe (MA)/LConn1 -- Exhaust/RConn1
  Thermal Resistor8/LConn1 -- Pipe (MA)/LConn2 -- Temperature Sensor/LConn1 -- Thermal Resistor/LConn1 -- Thermal Mass/LConn1 -- Thermal Resistor6/LConn1 -- Thermal Resistor7/LConn1 -- Thermal Resistor5/LConn1 -- Thermal Resistor4/LConn1 -- Thermal Resistor3/LConn1 -- Thermal Resistor1/LConn1
  PS-Simulink Converter5/LConn1 -- Pressure & Temperature Sensor (MA)1/RConn2
  PS-Simulink Converter4/LConn1 -- Pressure & Temperature Sensor (MA)1/RConn3
  Absolute Reference (MA)1/LConn1 -- Pressure & Temperature Sensor (MA)1/RConn1
